simulink model "psk8_pilot_phase_sync"  (Simulink 9.1)
settings: Solver=FixedStepDiscrete  StartTime=0.0  StopTime=inf  RelTol=1e-3
undefined symbols (not defined in the file): gcbh, i, rcfiltgaincompat
libraries: dspobslib x6, commfilt2 x2, commchan3 x1, commdigbbndpm3 x1, commrflib2 x1, commrandsrc2 x1, dspsigops x1
settings Model: Creator=Admin  LastModifiedBy=User
settings DataIOCC: LimitDataPoints=on  SignalLoggingSaveFormat=ModelDataLogs
settings OptimizationCC: ExpressionDepthLimit=2147483647  InitFltsAndDblsToZero=on
settings DebuggingCC: SolverPrmCheckMsg=warning  FcnCallInpInsideContextMsg=warning  StateNameClashWarn=warning

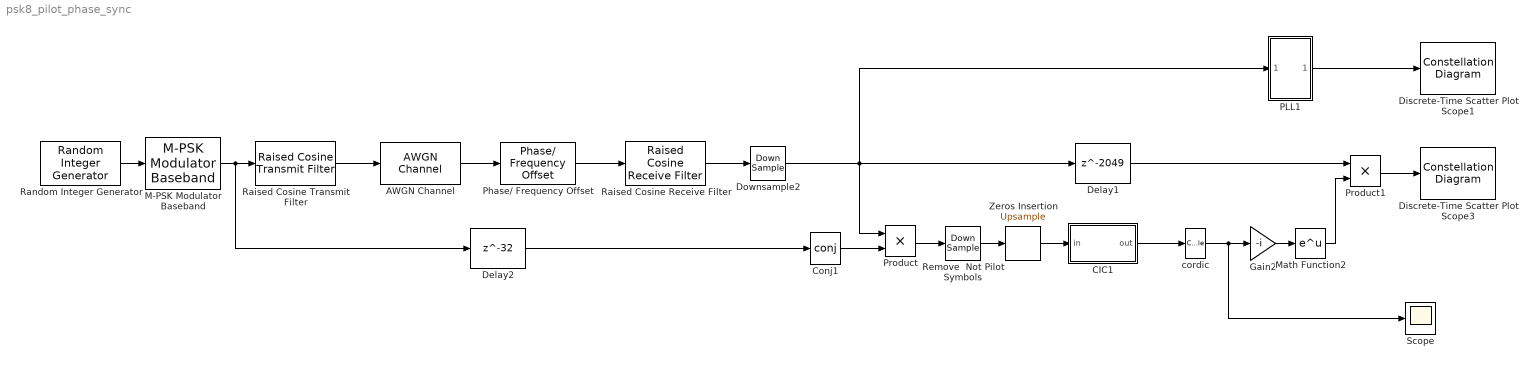
== system psk8_pilot_phase_sync ==
  AWGN Channel : commchan3/AWGN Channel  InputProcessing=Columns as channels (frame based)  seed=67  noiseMode="Signal to noise ratio  (Eb/No)"  EbNodB=12  EsNodB=10  SNRdB=10  bitsPerSym=2  Ps=0.1250  Tsym=1  variance=1
  CIC1 : Subsystem
  Conj1 : Math  Operator=conj  SaturateOnIntegerOverflow=on
  Delay1 : Delay  DelayLength=2049  InitialCondition=0  InputProcessing=Inherited
  Delay2 : Delay  DelayLength=32  InitialCondition=0  InputProcessing=Inherited
  Discrete-Time Scatter Plot Scope1 : ConstellationDiagram  Tag=ScatterPlot
  Discrete-Time Scatter Plot Scope3 : ConstellationDiagram  Tag=ScatterPlot
  Downsample2 : DownSample  N=8  InputProcessing=Inherited (this choice will be removed - see release notes)  RateOptions=Allow multirate processing
  Gain2 : Gain  Gain=-i  SaturateOnIntegerOverflow=on  OutDataTypeStr=Inherit: Same as input  ParamDataTypeStr=Inherit: Same as input
  M-PSK Modulator Baseband : commdigbbndpm3/M-PSK Modulator Baseband  M=8  InType=Integer  Enc=Gray  Mapping=[0:7]  Ph=0  outDtype=double  outWordLen=16  outUDDataType=sfix(16)  outFracLenMode=Best precision  outFracLen=15  outDataTypeStr=double  outLastDataTypeStr=double
      settings: SourceProductName=Communications System Toolbox
  Math Function2 : Math  SaturateOnIntegerOverflow=on
  PLL1 : Subsystem
  Phase/ Frequency Offset : commrflib2/Phase// Frequency Offset  phaseOffset=0  freqPort=off  freqOffset=1e-5
      settings: SourceProductName=Communications System Toolbox
  Product : Product
  Product1 : Product
  Raised Cosine Receive Filter : commfilt2/Raised Cosine Receive Filter  filtType=Square root  R=0.2  filtSpan=2*(16)  N=8  downFactor=1  downOffset=0  filterGain=rcfiltgaincompat(gcbh)  InputProcessing=Columns as channels (frame based)  RateOptions=Allow multirate processing  framing=Mute  checkCoeff=off  variableName=rcRxFilt  currentFiltSpan=2*(16)  D=16  inputOffset=0  sampMode=Mute  saveAsFlag=0  rateMode=Downsampling  checkGain=Normalized  launchFVT=off  roundingMode=Floor  overflowMode=off  coeffDataTypeStr=Inherit: Same word length as input  coeffMin=[]  coeffMax=[]  coeffLastDataTypeStr=Inherit: Same word length as input  accumDataTypeStr=Inherit: Same as product output  accumLastDataTypeStr=Inherit: Same as product output  outputDataTypeStr=Inherit: Same as accumulator  outputMin=[]  outputMax=[]  outputLastDataTypeStr=Inherit: Same as accumulator
  Raised Cosine Transmit Filter : commfilt2/Raised Cosine Transmit Filter  filtType=Square root  R=0.2  filtSpan=2*(16)  N=8  filterGain=rcfiltgaincompat(gcbh)  InputProcessing=Columns as channels (frame based)  RateOptions=Allow multirate processing  framing=Mute  checkCoeff=off  variableName=rcTxFilt  checkGain=Normalized  sampMode=Mute  saveAsFlag=0  currentFiltSpan=2*(16)  D=16  launchFVT=off  roundingMode=Floor  overflowMode=off  coeffDataTypeStr=Inherit: Same word length as input  coeffMin=[]  coeffMax=[]  coeffLastDataTypeStr=Inherit: Same word length as input  outputDataTypeStr=Inherit: Same as accumulator  outputMin=[]  outputMax=[]  outputLastDataTypeStr=Inherit: Same as accumulator
  Random Integer Generator : commrandsrc2/Random Integer Generator  mul=8  seed=37  Ts=1.  frameBased=off  sampPerFrame=1  orient=off  outDataType=double
  Remove  Not Pilot Symbols : DownSample  N=32  RateOptions=Allow multirate processing
  Scope : Scope
  Zeros Insertion : dspsigops/Upsample  N=32  phase=0  InputProcessing=Columns as channels (frame based)  RateOptions=Allow multirate processing  ic=0  mode=Unused parameter value
  cordic : ComplexToMagnitudeAngle  Output=Angle
  wires:
  Random Integer Generator/1 -> M-PSK Modulator Baseband/1
  M-PSK Modulator Baseband/1 -> Delay2/1, Raised Cosine Transmit Filter/1
  AWGN Channel/1 -> Phase/ Frequency Offset/1
  Phase/ Frequency Offset/1 -> Raised Cosine Receive Filter/1
  Product1/1 -> Discrete-Time Scatter Plot Scope3/1
  CIC1/1(out) -> cordic/1
  Delay1/1 -> Product1/1
  cordic/1 -> Scope/1, Gain2/1
  Gain2/1 -> Math Function2/1
  Math Function2/1 -> Product1/2
  Raised Cosine Receive Filter/1 -> Downsample2/1
  Product/1 -> Remove  Not Pilot Symbols/1
  Raised Cosine Transmit Filter/1 -> AWGN Channel/1
  Conj1/1 -> Product/2
  Delay2/1 -> Conj1/1
  Remove  Not Pilot Symbols/1 -> Zeros Insertion/1
  Zeros Insertion/1 -> CIC1/1(in)
  PLL1/1(Out1) -> Discrete-Time Scatter Plot Scope1/1
  Downsample2/1 -> PLL1/1(In1), Delay1/1, Product/1

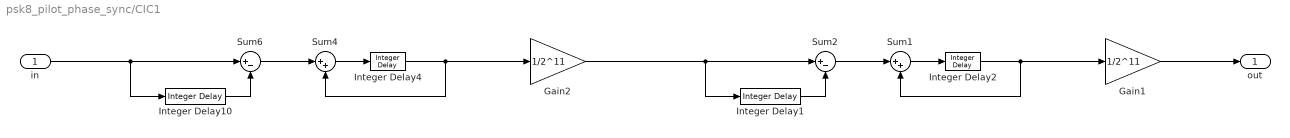
== system psk8_pilot_phase_sync/CIC1 ==
  in : Inport
  Gain1 : Gain  Gain=1/2^11  SaturateOnIntegerOverflow=on  OutDataTypeStr=Inherit: Same as input  ParamDataTypeStr=Inherit: Same as input
  Gain2 : Gain  Gain=1/2^11  SaturateOnIntegerOverflow=on  OutDataTypeStr=Inherit: Same as input  ParamDataTypeStr=Inherit: Same as input
  Integer Delay1 : dspobslib/Integer Delay  delay=2^11  ic=0  reset_popup=None
      settings: SourceProductName=DSP System Toolbox  SourceProductBaseCode=DS
  Integer Delay10 : dspobslib/Integer Delay  delay=2^11  ic=0  reset_popup=None
      settings: SourceProductName=DSP System Toolbox  SourceProductBaseCode=DS
  Integer Delay2 : dspobslib/Integer Delay  delay=1  ic=0  reset_popup=None
      settings: SourceProductName=DSP System Toolbox  SourceProductBaseCode=DS
  Integer Delay4 : dspobslib/Integer Delay  delay=1  ic=0  reset_popup=None
      settings: SourceProductName=DSP System Toolbox  SourceProductBaseCode=DS
  Sum1 : Sum  Inputs=|++  SaturateOnIntegerOverflow=on  InputSameDT=on  OutDataTypeStr=Inherit: Same as first input
  Sum2 : Sum  Inputs=|+-  SaturateOnIntegerOverflow=on  InputSameDT=on  OutDataTypeStr=Inherit: Same as first input
  Sum4 : Sum  Inputs=|++  SaturateOnIntegerOverflow=on  InputSameDT=on  OutDataTypeStr=Inherit: Same as first input
  Sum6 : Sum  Inputs=|+-  SaturateOnIntegerOverflow=on  InputSameDT=on  OutDataTypeStr=Inherit: Same as first input
  out : Outport
  wires:
  in/1 -> Sum6/1, Integer Delay10/1
  Integer Delay10/1 -> Sum6/2
  Sum4/1 -> Integer Delay4/1
  Integer Delay4/1 -> Sum4/2, Gain2/1
  Sum6/1 -> Sum4/1
  Sum2/1 -> Sum1/1
  Gain2/1 -> Sum2/1, Integer Delay1/1
  Sum1/1 -> Integer Delay2/1
  Integer Delay2/1 -> Sum1/2, Gain1/1
  Integer Delay1/1 -> Sum2/2
  Gain1/1 -> out/1

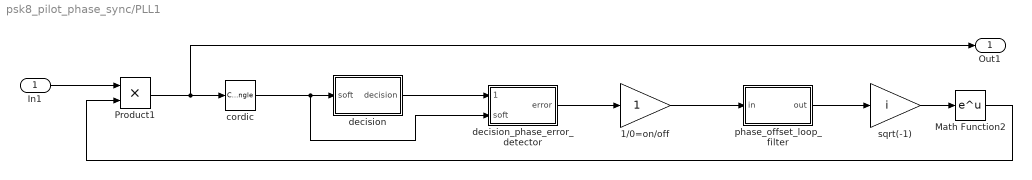
== system psk8_pilot_phase_sync/PLL1 ==
  In1 : Inport
  1/0=on/off : Gain  SaturateOnIntegerOverflow=on  OutDataTypeStr=Inherit: Same as input  ParamDataTypeStr=Inherit: Same as input
  Math Function2 : Math  OutputSignalType=complex  SaturateOnIntegerOverflow=on
  Product1 : Product  RndMeth=Zero
  cordic : ComplexToMagnitudeAngle  Output=Angle
  decision : Subsystem
  decision_phase_error_detector : Subsystem
  phase_offset_loop_filter : Subsystem
  sqrt(-1) : Gain  Gain=i  SaturateOnIntegerOverflow=on  OutDataTypeStr=Inherit: Same as input  ParamDataTypeStr=Inherit: Same as input
  Out1 : Outport
  wires:
  In1/1 -> Product1/1
  1/0=on/off/1 -> phase_offset_loop_filter/1(in)
  sqrt(-1)/1 -> Math Function2/1
  decision/1(decision) -> decision_phase_error_detector/1(decision)
  Product1/1 -> Out1/1, cordic/1
  phase_offset_loop_filter/1(out) -> sqrt(-1)/1
  cordic/1 -> decision/1(soft), decision_phase_error_detector/2(soft)
  Math Function2/1 -> Product1/2
  decision_phase_error_detector/1(error) -> 1/0=on/off/1

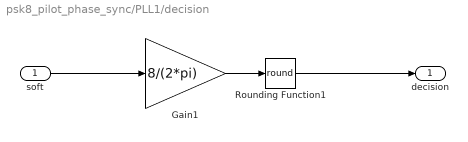
== system psk8_pilot_phase_sync/PLL1/decision ==
  soft : Inport
  Gain1 : Gain  Gain=8/(2*pi)  SaturateOnIntegerOverflow=on  OutDataTypeStr=Inherit: Same as input  ParamDataTypeStr=Inherit: Same as input
  Rounding Function1 : Rounding  Operator=round
  decision : Outport
  wires:
  soft/1 -> Gain1/1
  Gain1/1 -> Rounding Function1/1
  Rounding Function1/1 -> decision/1

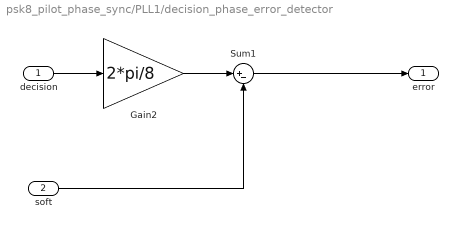
== system psk8_pilot_phase_sync/PLL1/decision_phase_error_detector ==
  decision : Inport
  soft : Inport  Port=2
  Gain2 : Gain  Gain=2*pi/8  SaturateOnIntegerOverflow=on  OutDataTypeStr=Inherit: Same as input  ParamDataTypeStr=Inherit: Same as input
  Sum1 : Sum  Inputs=|+-  SaturateOnIntegerOverflow=on
  error : Outport
  wires:
  decision/1 -> Gain2/1
  soft/1 -> Sum1/2
  Gain2/1 -> Sum1/1
  Sum1/1 -> error/1

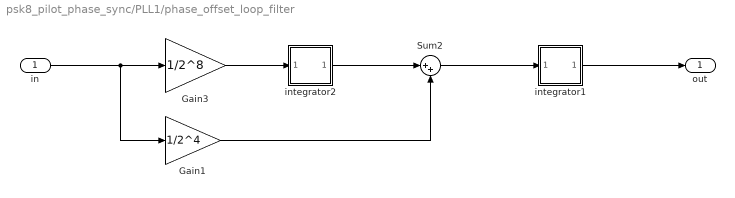
== system psk8_pilot_phase_sync/PLL1/phase_offset_loop_filter ==
  in : Inport
  Gain1 : Gain  Gain=1/2^4  SaturateOnIntegerOverflow=on  OutDataTypeStr=Inherit: Same as input  ParamDataTypeStr=Inherit: Same as input
  Gain3 : Gain  Gain=1/2^8  SaturateOnIntegerOverflow=on  OutDataTypeStr=Inherit: Same as input  ParamDataTypeStr=Inherit: Same as input
  Sum2 : Sum  Inputs=|++  SaturateOnIntegerOverflow=on  InputSameDT=on  OutDataTypeStr=Inherit: Same as first input
  integrator1 : Subsystem
  integrator2 : Subsystem
  out : Outport
  wires:
  Sum2/1 -> integrator1/1(In1)
  in/1 -> Gain3/1, Gain1/1
  Gain1/1 -> Sum2/2
  integrator1/1(Out1) -> out/1
  Gain3/1 -> integrator2/1(In1)
  integrator2/1(Out1) -> Sum2/1

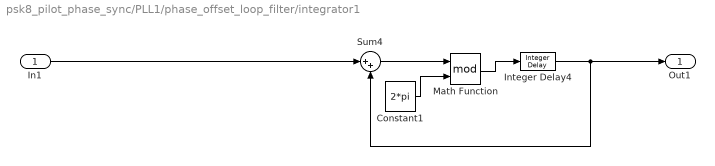
== system psk8_pilot_phase_sync/PLL1/phase_offset_loop_filter/integrator1 ==
  In1 : Inport
  Constant1 : Constant  Value=2*pi
  Integer Delay4 : dspobslib/Integer Delay  delay=1  ic=0  reset_popup=None
      settings: SourceProductName=DSP System Toolbox  SourceProductBaseCode=DS
  Math Function : Math  Operator=mod  SaturateOnIntegerOverflow=on
  Sum4 : Sum  Inputs=|++  SaturateOnIntegerOverflow=on  InputSameDT=on  OutDataTypeStr=Inherit: Same as first input
  Out1 : Outport
  wires:
  Sum4/1 -> Math Function/1
  Integer Delay4/1 -> Sum4/2, Out1/1
  In1/1 -> Sum4/1
  Math Function/1 -> Integer Delay4/1
  Constant1/1 -> Math Function/2

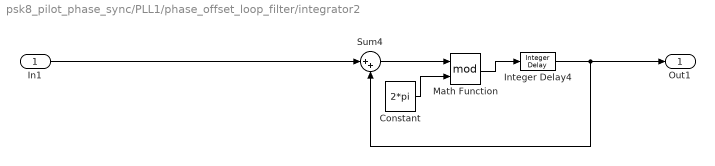
== system psk8_pilot_phase_sync/PLL1/phase_offset_loop_filter/integrator2 ==
  In1 : Inport
  Constant : Constant  Value=2*pi
  Integer Delay4 : dspobslib/Integer Delay  delay=1  ic=0  reset_popup=None
      settings: SourceProductName=DSP System Toolbox  SourceProductBaseCode=DS
  Math Function : Math  Operator=mod  SaturateOnIntegerOverflow=on
  Sum4 : Sum  Inputs=|++  SaturateOnIntegerOverflow=on  InputSameDT=on  OutDataTypeStr=Inherit: Same as first input
  Out1 : Outport
  wires:
  Sum4/1 -> Math Function/1
  Integer Delay4/1 -> Sum4/2, Out1/1
  In1/1 -> Sum4/1
  Math Function/1 -> Integer Delay4/1
  Constant/1 -> Math Function/2
